simulink model "artificial_algebraic_loops_GT"  (R2024b)
settings: Solver=VariableStepAuto  StartTime=0.0  StopTime=10.0  RelTol=1e-3
settings Model: Creator=xinxing  LastModifiedBy=xinxing

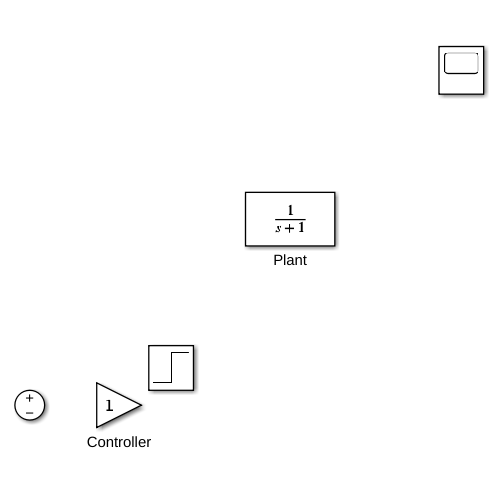
[thumbnail: Simulink's stored preview of the top-level diagram]
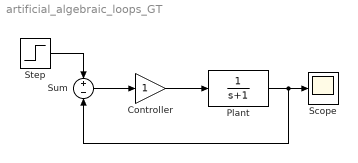
== system artificial_algebraic_loops_GT ==
  Controller : Gain
  Plant : TransferFcn  Denominator=[1 1]
  Scope : Scope
  Step : Step  SampleTime=0
  Sum : Sum  Inputs=+-
  wires:
  Plant/1 -> Scope/1, Sum/2
  Controller/1 -> Plant/1
  Sum/1 -> Controller/1
  Step/1 -> Sum/1
